simulink model "RoboticArmController"  (R2022a)
settings: Solver=VariableStepAuto  StartTime=0.0  StopTime=10.0  RelTol=1e-3
libraries: RAIP x1, RAOP x1
settings Model: Creator=shrey  LastModifiedBy=shrey

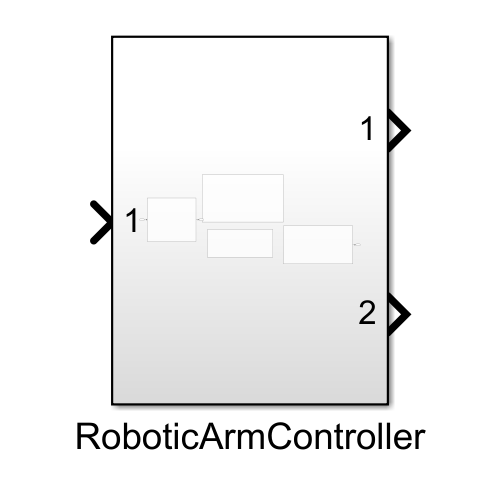
[thumbnail: Simulink's stored preview of the top-level diagram]
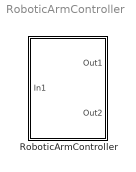
== system RoboticArmController ==
  RoboticArmController : Subsystem

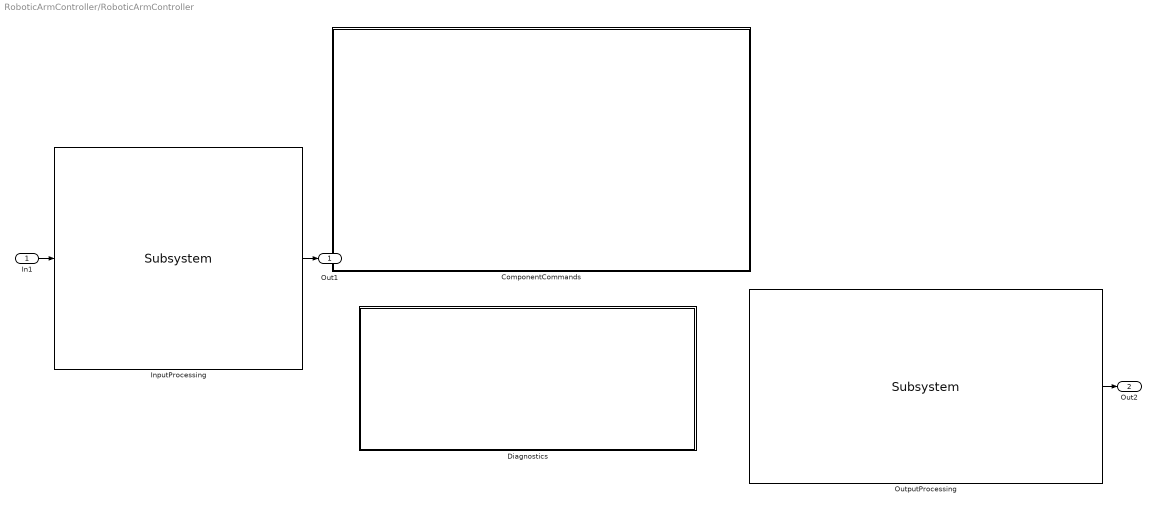
== system RoboticArmController/RoboticArmController ==
  In1 : Inport
  ComponentCommands : Subsystem
  Diagnostics : Subsystem
  InputProcessing : RAIP/Subsystem  SystemSampleTime=-1  VariantActivationTime=update diagram  Latency=0  AutoFrameSizeCalculation=off
  OutputProcessing : RAOP/Subsystem  SystemSampleTime=-1  VariantActivationTime=update diagram  Latency=0  AutoFrameSizeCalculation=off
  Out1 : Outport
  Out2 : Outport  Port=2
  wires:
  InputProcessing/1 -> Out1/1
  OutputProcessing/1 -> Out2/1
  In1/1 -> InputProcessing/1

== system RoboticArmController/RoboticArmController/ComponentCommands ==

== system RoboticArmController/RoboticArmController/Diagnostics ==
